simulink model "c00002M_harness"  (R2018a)
settings: Solver=FixedStepAuto  StartTime=0.0  StopTime=300  FixedStep=0.1  RelTol=1e-3
undefined symbols (not defined in the file): A1, hmax, R1, R2, sigbuilder_block, TempThreshold
(part 12 of 14)

== system c00002M_harness/M246/Tank3/Control ==
  note: 1: Maintenance
      | 2: Reference
      | 3: Manual
  ControlType : Inport
  ManualReference : Inport  Port=2
  EmergencyButton : Inport  Port=3
  Temperature : Inport  Port=4
  LiquidLevel : Inport  Port=5
  Constant : Constant  Value=0
  Constant1 : Constant  Value=TempThreshold
  Logical Operator : Logic  Operator=OR  AllPortsSameDT=off  OutDataTypeStr=boolean
  Logical Operator1 : Logic  Operator=OR  AllPortsSameDT=off  OutDataTypeStr=boolean
  ManualControlReference : Subsystem
  Relational Operator : RelationalOperator  Operator=>  OutDataTypeStr=boolean  RndMeth=Simplest
  Switch : Switch  Criteria=u2 > Threshold
  Switch1 : Switch  Criteria=u2 > Threshold
  LiquidIn : Outport
  LiquidOut : Outport  Port=2
  wires:
  ManualReference/1 -> ManualControlReference/1(ManualReference)
  LiquidLevel/1 -> ManualControlReference/2(LiquidLevel)
  Switch/1 -> LiquidIn/1
  Switch1/1 -> LiquidOut/1
  Constant/1 -> Switch1/1, Switch/1
  EmergencyButton/1 -> Logical Operator/1, Logical Operator1/1
  Relational Operator/1 -> Logical Operator1/2, Logical Operator/2
  Logical Operator/1 -> Switch1/2
  Logical Operator1/1 -> Switch/2
  Temperature/1 -> Relational Operator/1
  Constant1/1 -> Relational Operator/2
  ManualControlReference/1(LiquidIn) -> Switch/3
  ManualControlReference/2(LiquidOut) -> Switch1/3

== system c00002M_harness/M246/Tank3/TankModel ==
  LiquidIn : Inport
  LiquidOut : Inport  Port=2
  Add1 : Sum  Inputs=+-
  Constant1 : Constant  Value=0
  Constant2 : Constant  Value=0
  Constant3 : Constant
  Gain : Gain  Gain=1/R1
  Gain1 : Gain  Gain=1/A1
  Gain2 : Gain  Gain=1/R2
  Integrator : Integrator
  Saturation : Saturate  UpperLimit=hmax  LowerLimit=0
  Switch : Switch  Criteria=u2 ~= 0
  Switch1 : Switch  Criteria=u2 ~= 0
  LiquidLevel : Outport
  wires:
  Saturation/1 -> LiquidLevel/1, Gain2/1
  LiquidOut/1 -> Switch/2
  Add1/1 -> Gain1/1
  Gain2/1 -> Switch/1
  LiquidIn/1 -> Switch1/2
  Switch/1 -> Add1/2
  Switch1/1 -> Gain/1
  Constant2/1 -> Switch/3
  Constant3/1 -> Switch1/3
  Integrator/1 -> Saturation/1
  Gain1/1 -> Integrator/1
  Gain/1 -> Add1/1
  Constant1/1 -> Switch1/1

== system c00002M_harness/CPSUT/Tank1/Control/ManualControlReference ==
  ManualReference : Inport
  LiquidLevel : Inport  Port=2
  Add : Sum  Inputs=+-
  Add1 : Sum  Inputs=+-
  Gain1 : Gain  Gain=0.95
  Gain2 : Gain  Gain=0.95
  Relational Operator : RelationalOperator  Operator=>  OutDataTypeStr=boolean  RndMeth=Simplest
  Relational Operator1 : RelationalOperator  Operator=<  OutDataTypeStr=boolean  RndMeth=Simplest
  Saturation1 : Saturate  UpperLimit=hmax*0.9  LowerLimit=0
  LiquidIn : Outport
  LiquidOut : Outport  Port=2
  wires:
  LiquidLevel/1 -> Relational Operator/2, Add/1, Add1/1, Gain2/1
  Relational Operator/1 -> LiquidIn/1
  Relational Operator1/1 -> LiquidOut/1
  Add/1 -> Add1/2
  Add1/1 -> Relational Operator1/2
  Gain1/1 -> Saturation1/1
  Gain2/1 -> Add/2
  ManualReference/1 -> Gain1/1
  Saturation1/1 -> Relational Operator1/1, Relational Operator/1

== system c00002M_harness/CPSUT/Tank3/Control/ManualControlReference ==
  ManualReference : Inport
  LiquidLevel : Inport  Port=2
  Add : Sum  Inputs=+-
  Add1 : Sum  Inputs=+-
  Gain1 : Gain  Gain=0.95
  Gain2 : Gain  Gain=0.95
  Relational Operator : RelationalOperator  Operator=>  OutDataTypeStr=boolean  RndMeth=Simplest
  Relational Operator1 : RelationalOperator  Operator=<  OutDataTypeStr=boolean  RndMeth=Simplest
  Saturation1 : Saturate  UpperLimit=hmax*0.9  LowerLimit=0
  LiquidIn : Outport
  LiquidOut : Outport  Port=2
  wires:
  LiquidLevel/1 -> Relational Operator/2, Add/1, Add1/1, Gain2/1
  Relational Operator/1 -> LiquidIn/1
  Relational Operator1/1 -> LiquidOut/1
  Add/1 -> Add1/2
  Add1/1 -> Relational Operator1/2
  Gain1/1 -> Saturation1/1
  Gain2/1 -> Add/2
  ManualReference/1 -> Gain1/1
  Saturation1/1 -> Relational Operator1/1, Relational Operator/1

== system c00002M_harness/M001/Tank1/Control/ManualControlReference ==
  ManualReference : Inport
  LiquidLevel : Inport  Port=2
  Add : Sum  Inputs=+-
  Add1 : Sum  Inputs=+-
  Gain1 : Gain  Gain=0.95
  Gain2 : Gain  Gain=0.95
  Relational Operator : RelationalOperator  Operator=>  OutDataTypeStr=boolean  RndMeth=Simplest
  Relational Operator1 : RelationalOperator  Operator=<  OutDataTypeStr=boolean  RndMeth=Simplest
  Saturation1 : Saturate  UpperLimit=hmax*0.9  LowerLimit=0
  LiquidIn : Outport
  LiquidOut : Outport  Port=2
  wires:
  Saturation1/1 -> Relational Operator/1, Relational Operator1/1
  ManualReference/1 -> Gain1/1
  Gain2/1 -> Add/2
  Gain1/1 -> Saturation1/1
  Add1/1 -> Relational Operator1/2
  Add/1 -> Add1/2
  Relational Operator1/1 -> LiquidOut/1
  Relational Operator/1 -> LiquidIn/1
  LiquidLevel/1 -> Gain2/1, Add1/1, Add/1, Relational Operator/2

== system c00002M_harness/M001/Tank3/Control/ManualControlReference ==
  ManualReference : Inport
  LiquidLevel : Inport  Port=2
  Add : Sum  Inputs=+-
  Add1 : Sum  Inputs=+-
  Gain1 : Gain  Gain=0.95
  Gain2 : Gain  Gain=0.95
  Relational Operator : RelationalOperator  Operator=>  OutDataTypeStr=boolean  RndMeth=Simplest
  Relational Operator1 : RelationalOperator  Operator=<  OutDataTypeStr=boolean  RndMeth=Simplest
  Saturation1 : Saturate  UpperLimit=hmax*0.9  LowerLimit=0
  LiquidIn : Outport
  LiquidOut : Outport  Port=2
  wires:
  Saturation1/1 -> Relational Operator/1, Relational Operator1/1
  ManualReference/1 -> Gain1/1
  Gain2/1 -> Add/2
  Gain1/1 -> Saturation1/1
  Add1/1 -> Relational Operator1/2
  Add/1 -> Add1/2
  Relational Operator1/1 -> LiquidOut/1
  Relational Operator/1 -> LiquidIn/1
  LiquidLevel/1 -> Gain2/1, Add1/1, Add/1, Relational Operator/2

== system c00002M_harness/M002/Tank1/Control/ManualControlReference ==
  ManualReference : Inport
  LiquidLevel : Inport  Port=2
  Add : Sum  Inputs=+-
  Add1 : Sum  Inputs=+-
  Gain1 : Gain  Gain=0.95
  Gain2 : Gain  Gain=0.95
  Relational Operator : RelationalOperator  Operator=>  OutDataTypeStr=boolean  RndMeth=Simplest
  Relational Operator1 : RelationalOperator  Operator=<  OutDataTypeStr=boolean  RndMeth=Simplest
  Saturation1 : Saturate  UpperLimit=hmax*0.9  LowerLimit=0
  LiquidIn : Outport
  LiquidOut : Outport  Port=2
  wires:
  LiquidLevel/1 -> Relational Operator/2, Add/1, Add1/1, Gain2/1
  Relational Operator/1 -> LiquidIn/1
  Relational Operator1/1 -> LiquidOut/1
  Add/1 -> Add1/2
  Add1/1 -> Relational Operator1/2
  Gain1/1 -> Saturation1/1
  Gain2/1 -> Add/2
  ManualReference/1 -> Gain1/1
  Saturation1/1 -> Relational Operator1/1, Relational Operator/1

== system c00002M_harness/M002/Tank3/Control/ManualControlReference ==
  ManualReference : Inport
  LiquidLevel : Inport  Port=2
  Add : Sum  Inputs=+-
  Add1 : Sum  Inputs=+-
  Gain1 : Gain  Gain=0.95
  Gain2 : Gain  Gain=0.95
  Relational Operator : RelationalOperator  Operator=>  OutDataTypeStr=boolean  RndMeth=Simplest
  Relational Operator1 : RelationalOperator  Operator=<  OutDataTypeStr=boolean  RndMeth=Simplest
  Saturation1 : Saturate  UpperLimit=hmax*0.9  LowerLimit=0
  LiquidIn : Outport
  LiquidOut : Outport  Port=2
  wires:
  LiquidLevel/1 -> Relational Operator/2, Add/1, Add1/1, Gain2/1
  Relational Operator/1 -> LiquidIn/1
  Relational Operator1/1 -> LiquidOut/1
  Add/1 -> Add1/2
  Add1/1 -> Relational Operator1/2
  Gain1/1 -> Saturation1/1
  Gain2/1 -> Add/2
  ManualReference/1 -> Gain1/1
  Saturation1/1 -> Relational Operator1/1, Relational Operator/1

== system c00002M_harness/M003/Tank1/Control/ManualControlReference ==
  ManualReference : Inport
  LiquidLevel : Inport  Port=2
  Add : Sum  Inputs=+-
  Add1 : Sum  Inputs=+-
  Gain1 : Gain  Gain=0.95
  Gain2 : Gain  Gain=0.95
  Relational Operator : RelationalOperator  Operator=>  OutDataTypeStr=boolean  RndMeth=Simplest
  Relational Operator1 : RelationalOperator  Operator=<  OutDataTypeStr=boolean  RndMeth=Simplest
  Saturation1 : Saturate  UpperLimit=hmax*0.9  LowerLimit=0
  LiquidIn : Outport
  LiquidOut : Outport  Port=2
  wires:
  LiquidLevel/1 -> Relational Operator/2, Add/1, Add1/1, Gain2/1
  Relational Operator/1 -> LiquidIn/1
  Relational Operator1/1 -> LiquidOut/1
  Add/1 -> Add1/2
  Add1/1 -> Relational Operator1/2
  Gain1/1 -> Saturation1/1
  Gain2/1 -> Add/2
  ManualReference/1 -> Gain1/1
  Saturation1/1 -> Relational Operator1/1, Relational Operator/1

== system c00002M_harness/M003/Tank3/Control/ManualControlReference ==
  ManualReference : Inport
  LiquidLevel : Inport  Port=2
  Add : Sum  Inputs=+-
  Add1 : Sum  Inputs=+-
  Gain1 : Gain  Gain=0.95
  Gain2 : Gain  Gain=0.95
  Relational Operator : RelationalOperator  Operator=>  OutDataTypeStr=boolean  RndMeth=Simplest
  Relational Operator1 : RelationalOperator  Operator=<  OutDataTypeStr=boolean  RndMeth=Simplest
  Saturation1 : Saturate  UpperLimit=hmax*0.9  LowerLimit=0
  LiquidIn : Outport
  LiquidOut : Outport  Port=2
  wires:
  LiquidLevel/1 -> Relational Operator/2, Add/1, Add1/1, Gain2/1
  Relational Operator/1 -> LiquidIn/1
  Relational Operator1/1 -> LiquidOut/1
  Add/1 -> Add1/2
  Add1/1 -> Relational Operator1/2
  Gain1/1 -> Saturation1/1
  Gain2/1 -> Add/2
  ManualReference/1 -> Gain1/1
  Saturation1/1 -> Relational Operator1/1, Relational Operator/1

== system c00002M_harness/M004/Tank1/Control/ManualControlReference ==
  ManualReference : Inport
  LiquidLevel : Inport  Port=2
  Add : Sum  Inputs=+-
  Add1 : Sum  Inputs=+-
  Gain1 : Gain  Gain=0.95
  Gain2 : Gain  Gain=0.95
  Relational Operator : RelationalOperator  Operator=>  OutDataTypeStr=boolean  RndMeth=Simplest
  Relational Operator1 : RelationalOperator  Operator=<  OutDataTypeStr=boolean  RndMeth=Simplest
  Saturation1 : Saturate  UpperLimit=hmax*0.9  LowerLimit=0
  LiquidIn : Outport
  LiquidOut : Outport  Port=2
  wires:
  LiquidLevel/1 -> Relational Operator/2, Add/1, Add1/1, Gain2/1
  Relational Operator/1 -> LiquidIn/1
  Relational Operator1/1 -> LiquidOut/1
  Add/1 -> Add1/2
  Add1/1 -> Relational Operator1/2
  Gain1/1 -> Saturation1/1
  Gain2/1 -> Add/2
  ManualReference/1 -> Gain1/1
  Saturation1/1 -> Relational Operator1/1, Relational Operator/1

== system c00002M_harness/M004/Tank3/Control/ManualControlReference ==
  ManualReference : Inport
  LiquidLevel : Inport  Port=2
  Add : Sum  Inputs=+-
  Add1 : Sum  Inputs=+-
  Gain1 : Gain  Gain=0.95
  Gain2 : Gain  Gain=0.95
  Relational Operator : RelationalOperator  Operator=>  OutDataTypeStr=boolean  RndMeth=Simplest
  Relational Operator1 : RelationalOperator  Operator=<  OutDataTypeStr=boolean  RndMeth=Simplest
  Saturation1 : Saturate  UpperLimit=hmax*0.9  LowerLimit=0
  LiquidIn : Outport
  LiquidOut : Outport  Port=2
  wires:
  LiquidLevel/1 -> Relational Operator/2, Add/1, Add1/1, Gain2/1
  Relational Operator/1 -> LiquidIn/1
  Relational Operator1/1 -> LiquidOut/1
  Add/1 -> Add1/2
  Add1/1 -> Relational Operator1/2
  Gain1/1 -> Saturation1/1
  Gain2/1 -> Add/2
  ManualReference/1 -> Gain1/1
  Saturation1/1 -> Relational Operator1/1, Relational Operator/1

== system c00002M_harness/M046/Tank1/Control/ManualControlReference ==
  ManualReference : Inport
  LiquidLevel : Inport  Port=2
  Add : Sum
  Add1 : Sum  Inputs=+-
  Gain1 : Gain  Gain=0.95
  Gain2 : Gain  Gain=0.95
  Relational Operator : RelationalOperator  Operator=>  OutDataTypeStr=boolean  RndMeth=Simplest
  Relational Operator1 : RelationalOperator  Operator=<  OutDataTypeStr=boolean  RndMeth=Simplest
  Saturation1 : Saturate  UpperLimit=hmax*0.9  LowerLimit=0
  LiquidIn : Outport
  LiquidOut : Outport  Port=2
  wires:
  LiquidLevel/1 -> Relational Operator/2, Add/1, Add1/1, Gain2/1
  Relational Operator/1 -> LiquidIn/1
  Relational Operator1/1 -> LiquidOut/1
  Add/1 -> Add1/2
  Add1/1 -> Relational Operator1/2
  Gain1/1 -> Saturation1/1
  Gain2/1 -> Add/2
  ManualReference/1 -> Gain1/1
  Saturation1/1 -> Relational Operator1/1, Relational Operator/1

== system c00002M_harness/M046/Tank3/Control/ManualControlReference ==
  ManualReference : Inport
  LiquidLevel : Inport  Port=2
  Add : Sum  Inputs=+-
  Add1 : Sum  Inputs=+-
  Gain1 : Gain  Gain=0.95
  Gain2 : Gain  Gain=0.95
  Relational Operator : RelationalOperator  Operator=>  OutDataTypeStr=boolean  RndMeth=Simplest
  Relational Operator1 : RelationalOperator  Operator=<  OutDataTypeStr=boolean  RndMeth=Simplest
  Saturation1 : Saturate  UpperLimit=hmax*0.9  LowerLimit=0
  LiquidIn : Outport
  LiquidOut : Outport  Port=2
  wires:
  LiquidLevel/1 -> Relational Operator/2, Add/1, Add1/1, Gain2/1
  Relational Operator/1 -> LiquidIn/1
  Relational Operator1/1 -> LiquidOut/1
  Add/1 -> Add1/2
  Add1/1 -> Relational Operator1/2
  Gain1/1 -> Saturation1/1
  Gain2/1 -> Add/2
  ManualReference/1 -> Gain1/1
  Saturation1/1 -> Relational Operator1/1, Relational Operator/1

== system c00002M_harness/M047/Tank1/Control/ManualControlReference ==
  ManualReference : Inport
  LiquidLevel : Inport  Port=2
  Add : Sum  Inputs=--
  Add1 : Sum  Inputs=+-
  Gain1 : Gain  Gain=0.95
  Gain2 : Gain  Gain=0.95
  Relational Operator : RelationalOperator  Operator=>  OutDataTypeStr=boolean  RndMeth=Simplest
  Relational Operator1 : RelationalOperator  Operator=<  OutDataTypeStr=boolean  RndMeth=Simplest
  Saturation1 : Saturate  UpperLimit=hmax*0.9  LowerLimit=0
  LiquidIn : Outport
  LiquidOut : Outport  Port=2
  wires:
  LiquidLevel/1 -> Relational Operator/2, Add/1, Add1/1, Gain2/1
  Relational Operator/1 -> LiquidIn/1
  Relational Operator1/1 -> LiquidOut/1
  Add/1 -> Add1/2
  Add1/1 -> Relational Operator1/2
  Gain1/1 -> Saturation1/1
  Gain2/1 -> Add/2
  ManualReference/1 -> Gain1/1
  Saturation1/1 -> Relational Operator1/1, Relational Operator/1

== system c00002M_harness/M047/Tank3/Control/ManualControlReference ==
  ManualReference : Inport
  LiquidLevel : Inport  Port=2
  Add : Sum  Inputs=+-
  Add1 : Sum  Inputs=+-
  Gain1 : Gain  Gain=0.95
  Gain2 : Gain  Gain=0.95
  Relational Operator : RelationalOperator  Operator=>  OutDataTypeStr=boolean  RndMeth=Simplest
  Relational Operator1 : RelationalOperator  Operator=<  OutDataTypeStr=boolean  RndMeth=Simplest
  Saturation1 : Saturate  UpperLimit=hmax*0.9  LowerLimit=0
  LiquidIn : Outport
  LiquidOut : Outport  Port=2
  wires:
  LiquidLevel/1 -> Relational Operator/2, Add/1, Add1/1, Gain2/1
  Relational Operator/1 -> LiquidIn/1
  Relational Operator1/1 -> LiquidOut/1
  Add/1 -> Add1/2
  Add1/1 -> Relational Operator1/2
  Gain1/1 -> Saturation1/1
  Gain2/1 -> Add/2
  ManualReference/1 -> Gain1/1
  Saturation1/1 -> Relational Operator1/1, Relational Operator/1

== system c00002M_harness/M048/Tank1/Control/ManualControlReference ==
  ManualReference : Inport
  LiquidLevel : Inport  Port=2
  Add : Sum  Inputs=-+
  Add1 : Sum  Inputs=+-
  Gain1 : Gain  Gain=0.95
  Gain2 : Gain  Gain=0.95
  Relational Operator : RelationalOperator  Operator=>  OutDataTypeStr=boolean  RndMeth=Simplest
  Relational Operator1 : RelationalOperator  Operator=<  OutDataTypeStr=boolean  RndMeth=Simplest
  Saturation1 : Saturate  UpperLimit=hmax*0.9  LowerLimit=0
  LiquidIn : Outport
  LiquidOut : Outport  Port=2
  wires:
  LiquidLevel/1 -> Relational Operator/2, Add/1, Add1/1, Gain2/1
  Relational Operator/1 -> LiquidIn/1
  Relational Operator1/1 -> LiquidOut/1
  Add/1 -> Add1/2
  Add1/1 -> Relational Operator1/2
  Gain1/1 -> Saturation1/1
  Gain2/1 -> Add/2
  ManualReference/1 -> Gain1/1
  Saturation1/1 -> Relational Operator1/1, Relational Operator/1

== system c00002M_harness/M048/Tank3/Control/ManualControlReference ==
  ManualReference : Inport
  LiquidLevel : Inport  Port=2
  Add : Sum  Inputs=+-
  Add1 : Sum  Inputs=+-
  Gain1 : Gain  Gain=0.95
  Gain2 : Gain  Gain=0.95
  Relational Operator : RelationalOperator  Operator=>  OutDataTypeStr=boolean  RndMeth=Simplest
  Relational Operator1 : RelationalOperator  Operator=<  OutDataTypeStr=boolean  RndMeth=Simplest
  Saturation1 : Saturate  UpperLimit=hmax*0.9  LowerLimit=0
  LiquidIn : Outport
  LiquidOut : Outport  Port=2
  wires:
  LiquidLevel/1 -> Relational Operator/2, Add/1, Add1/1, Gain2/1
  Relational Operator/1 -> LiquidIn/1
  Relational Operator1/1 -> LiquidOut/1
  Add/1 -> Add1/2
  Add1/1 -> Relational Operator1/2
  Gain1/1 -> Saturation1/1
  Gain2/1 -> Add/2
  ManualReference/1 -> Gain1/1
  Saturation1/1 -> Relational Operator1/1, Relational Operator/1

== system c00002M_harness/M049/Tank1/Control/ManualControlReference ==
  ManualReference : Inport
  LiquidLevel : Inport  Port=2
  Add : Sum  Inputs=+-
  Add1 : Sum
  Gain1 : Gain  Gain=0.95
  Gain2 : Gain  Gain=0.95
  Relational Operator : RelationalOperator  Operator=>  OutDataTypeStr=boolean  RndMeth=Simplest
  Relational Operator1 : RelationalOperator  Operator=<  OutDataTypeStr=boolean  RndMeth=Simplest
  Saturation1 : Saturate  UpperLimit=hmax*0.9  LowerLimit=0
  LiquidIn : Outport
  LiquidOut : Outport  Port=2
  wires:
  LiquidLevel/1 -> Relational Operator/2, Add/1, Add1/1, Gain2/1
  Relational Operator/1 -> LiquidIn/1
  Relational Operator1/1 -> LiquidOut/1
  Add/1 -> Add1/2
  Add1/1 -> Relational Operator1/2
  Gain1/1 -> Saturation1/1
  Gain2/1 -> Add/2
  ManualReference/1 -> Gain1/1
  Saturation1/1 -> Relational Operator1/1, Relational Operator/1

== system c00002M_harness/M049/Tank3/Control/ManualControlReference ==
  ManualReference : Inport
  LiquidLevel : Inport  Port=2
  Add : Sum  Inputs=+-
  Add1 : Sum  Inputs=+-
  Gain1 : Gain  Gain=0.95
  Gain2 : Gain  Gain=0.95
  Relational Operator : RelationalOperator  Operator=>  OutDataTypeStr=boolean  RndMeth=Simplest
  Relational Operator1 : RelationalOperator  Operator=<  OutDataTypeStr=boolean  RndMeth=Simplest
  Saturation1 : Saturate  UpperLimit=hmax*0.9  LowerLimit=0
  LiquidIn : Outport
  LiquidOut : Outport  Port=2
  wires:
  LiquidLevel/1 -> Relational Operator/2, Add/1, Add1/1, Gain2/1
  Relational Operator/1 -> LiquidIn/1
  Relational Operator1/1 -> LiquidOut/1
  Add/1 -> Add1/2
  Add1/1 -> Relational Operator1/2
  Gain1/1 -> Saturation1/1
  Gain2/1 -> Add/2
  ManualReference/1 -> Gain1/1
  Saturation1/1 -> Relational Operator1/1, Relational Operator/1

== system c00002M_harness/M050/Tank1/Control/ManualControlReference ==
  ManualReference : Inport
  LiquidLevel : Inport  Port=2
  Add : Sum  Inputs=+-
  Add1 : Sum  Inputs=--
  Gain1 : Gain  Gain=0.95
  Gain2 : Gain  Gain=0.95
  Relational Operator : RelationalOperator  Operator=>  OutDataTypeStr=boolean  RndMeth=Simplest
  Relational Operator1 : RelationalOperator  Operator=<  OutDataTypeStr=boolean  RndMeth=Simplest
  Saturation1 : Saturate  UpperLimit=hmax*0.9  LowerLimit=0
  LiquidIn : Outport
  LiquidOut : Outport  Port=2
  wires:
  LiquidLevel/1 -> Relational Operator/2, Add/1, Add1/1, Gain2/1
  Relational Operator/1 -> LiquidIn/1
  Relational Operator1/1 -> LiquidOut/1
  Add/1 -> Add1/2
  Add1/1 -> Relational Operator1/2
  Gain1/1 -> Saturation1/1
  Gain2/1 -> Add/2
  ManualReference/1 -> Gain1/1
  Saturation1/1 -> Relational Operator1/1, Relational Operator/1

== system c00002M_harness/M050/Tank3/Control/ManualControlReference ==
  ManualReference : Inport
  LiquidLevel : Inport  Port=2
  Add : Sum  Inputs=+-
  Add1 : Sum  Inputs=+-
  Gain1 : Gain  Gain=0.95
  Gain2 : Gain  Gain=0.95
  Relational Operator : RelationalOperator  Operator=>  OutDataTypeStr=boolean  RndMeth=Simplest
  Relational Operator1 : RelationalOperator  Operator=<  OutDataTypeStr=boolean  RndMeth=Simplest
  Saturation1 : Saturate  UpperLimit=hmax*0.9  LowerLimit=0
  LiquidIn : Outport
  LiquidOut : Outport  Port=2
  wires:
  LiquidLevel/1 -> Relational Operator/2, Add/1, Add1/1, Gain2/1
  Relational Operator/1 -> LiquidIn/1
  Relational Operator1/1 -> LiquidOut/1
  Add/1 -> Add1/2
  Add1/1 -> Relational Operator1/2
  Gain1/1 -> Saturation1/1
  Gain2/1 -> Add/2
  ManualReference/1 -> Gain1/1
  Saturation1/1 -> Relational Operator1/1, Relational Operator/1

== system c00002M_harness/M051/Tank1/Control/ManualControlReference ==
  ManualReference : Inport
  LiquidLevel : Inport  Port=2
  Add : Sum  Inputs=+-
  Add1 : Sum  Inputs=-+
  Gain1 : Gain  Gain=0.95
  Gain2 : Gain  Gain=0.95
  Relational Operator : RelationalOperator  Operator=>  OutDataTypeStr=boolean  RndMeth=Simplest
  Relational Operator1 : RelationalOperator  Operator=<  OutDataTypeStr=boolean  RndMeth=Simplest
  Saturation1 : Saturate  UpperLimit=hmax*0.9  LowerLimit=0
  LiquidIn : Outport
  LiquidOut : Outport  Port=2
  wires:
  LiquidLevel/1 -> Relational Operator/2, Add/1, Add1/1, Gain2/1
  Relational Operator/1 -> LiquidIn/1
  Relational Operator1/1 -> LiquidOut/1
  Add/1 -> Add1/2
  Add1/1 -> Relational Operator1/2
  Gain1/1 -> Saturation1/1
  Gain2/1 -> Add/2
  ManualReference/1 -> Gain1/1
  Saturation1/1 -> Relational Operator1/1, Relational Operator/1

== system c00002M_harness/M051/Tank3/Control/ManualControlReference ==
  ManualReference : Inport
  LiquidLevel : Inport  Port=2
  Add : Sum  Inputs=+-
  Add1 : Sum  Inputs=+-
  Gain1 : Gain  Gain=0.95
  Gain2 : Gain  Gain=0.95
  Relational Operator : RelationalOperator  Operator=>  OutDataTypeStr=boolean  RndMeth=Simplest
  Relational Operator1 : RelationalOperator  Operator=<  OutDataTypeStr=boolean  RndMeth=Simplest
  Saturation1 : Saturate  UpperLimit=hmax*0.9  LowerLimit=0
  LiquidIn : Outport
  LiquidOut : Outport  Port=2
  wires:
  LiquidLevel/1 -> Relational Operator/2, Add/1, Add1/1, Gain2/1
  Relational Operator/1 -> LiquidIn/1
  Relational Operator1/1 -> LiquidOut/1
  Add/1 -> Add1/2
  Add1/1 -> Relational Operator1/2
  Gain1/1 -> Saturation1/1
  Gain2/1 -> Add/2
  ManualReference/1 -> Gain1/1
  Saturation1/1 -> Relational Operator1/1, Relational Operator/1

== system c00002M_harness/M052/Tank1/Control/ManualControlReference ==
  ManualReference : Inport
  LiquidLevel : Inport  Port=2
  Add : Sum  Inputs=+-
  Add1 : Sum  Inputs=+-
  Gain1 : Gain  Gain=0.90
  Gain2 : Gain  Gain=0.95
  Relational Operator : RelationalOperator  Operator=>  OutDataTypeStr=boolean  RndMeth=Simplest
  Relational Operator1 : RelationalOperator  Operator=<  OutDataTypeStr=boolean  RndMeth=Simplest
  Saturation1 : Saturate  UpperLimit=hmax*0.9  LowerLimit=0
  LiquidIn : Outport
  LiquidOut : Outport  Port=2
  wires:
  LiquidLevel/1 -> Relational Operator/2, Add/1, Add1/1, Gain2/1
  Relational Operator/1 -> LiquidIn/1
  Relational Operator1/1 -> LiquidOut/1
  Add/1 -> Add1/2
  Add1/1 -> Relational Operator1/2
  Gain1/1 -> Saturation1/1
  Gain2/1 -> Add/2
  ManualReference/1 -> Gain1/1
  Saturation1/1 -> Relational Operator1/1, Relational Operator/1

== system c00002M_harness/M052/Tank3/Control/ManualControlReference ==
  ManualReference : Inport
  LiquidLevel : Inport  Port=2
  Add : Sum  Inputs=+-
  Add1 : Sum  Inputs=+-
  Gain1 : Gain  Gain=0.95
  Gain2 : Gain  Gain=0.95
  Relational Operator : RelationalOperator  Operator=>  OutDataTypeStr=boolean  RndMeth=Simplest
  Relational Operator1 : RelationalOperator  Operator=<  OutDataTypeStr=boolean  RndMeth=Simplest
  Saturation1 : Saturate  UpperLimit=hmax*0.9  LowerLimit=0
  LiquidIn : Outport
  LiquidOut : Outport  Port=2
  wires:
  LiquidLevel/1 -> Relational Operator/2, Add/1, Add1/1, Gain2/1
  Relational Operator/1 -> LiquidIn/1
  Relational Operator1/1 -> LiquidOut/1
  Add/1 -> Add1/2
  Add1/1 -> Relational Operator1/2
  Gain1/1 -> Saturation1/1
  Gain2/1 -> Add/2
  ManualReference/1 -> Gain1/1
  Saturation1/1 -> Relational Operator1/1, Relational Operator/1

== system c00002M_harness/M053/Tank1/Control/ManualControlReference ==
  ManualReference : Inport
  LiquidLevel : Inport  Port=2
  Add : Sum  Inputs=+-
  Add1 : Sum  Inputs=+-
  Gain1 : Gain  Gain=0.95
  Gain2 : Gain  Gain=0.90
  Relational Operator : RelationalOperator  Operator=>  OutDataTypeStr=boolean  RndMeth=Simplest
  Relational Operator1 : RelationalOperator  Operator=<  OutDataTypeStr=boolean  RndMeth=Simplest
  Saturation1 : Saturate  UpperLimit=hmax*0.9  LowerLimit=0
  LiquidIn : Outport
  LiquidOut : Outport  Port=2
  wires:
  LiquidLevel/1 -> Relational Operator/2, Add/1, Add1/1, Gain2/1
  Relational Operator/1 -> LiquidIn/1
  Relational Operator1/1 -> LiquidOut/1
  Add/1 -> Add1/2
  Add1/1 -> Relational Operator1/2
  Gain1/1 -> Saturation1/1
  Gain2/1 -> Add/2
  ManualReference/1 -> Gain1/1
  Saturation1/1 -> Relational Operator1/1, Relational Operator/1

== system c00002M_harness/M053/Tank3/Control/ManualControlReference ==
  ManualReference : Inport
  LiquidLevel : Inport  Port=2
  Add : Sum  Inputs=+-
  Add1 : Sum  Inputs=+-
  Gain1 : Gain  Gain=0.95
  Gain2 : Gain  Gain=0.95
  Relational Operator : RelationalOperator  Operator=>  OutDataTypeStr=boolean  RndMeth=Simplest
  Relational Operator1 : RelationalOperator  Operator=<  OutDataTypeStr=boolean  RndMeth=Simplest
  Saturation1 : Saturate  UpperLimit=hmax*0.9  LowerLimit=0
  LiquidIn : Outport
  LiquidOut : Outport  Port=2
  wires:
  LiquidLevel/1 -> Relational Operator/2, Add/1, Add1/1, Gain2/1
  Relational Operator/1 -> LiquidIn/1
  Relational Operator1/1 -> LiquidOut/1
  Add/1 -> Add1/2
  Add1/1 -> Relational Operator1/2
  Gain1/1 -> Saturation1/1
  Gain2/1 -> Add/2
  ManualReference/1 -> Gain1/1
  Saturation1/1 -> Relational Operator1/1, Relational Operator/1

== system c00002M_harness/M054/Tank1/Control/ManualControlReference ==
  ManualReference : Inport
  LiquidLevel : Inport  Port=2
  Add : Sum  Inputs=+-
  Add1 : Sum  Inputs=+-
  Gain1 : Gain  Gain=0.95
  Gain2 : Gain  Gain=0.95
  Relational Operator : RelationalOperator  Operator=<  OutDataTypeStr=boolean  RndMeth=Simplest
  Relational Operator1 : RelationalOperator  Operator=<  OutDataTypeStr=boolean  RndMeth=Simplest
  Saturation1 : Saturate  UpperLimit=hmax*0.9  LowerLimit=0
  LiquidIn : Outport
  LiquidOut : Outport  Port=2
  wires:
  LiquidLevel/1 -> Relational Operator/2, Add/1, Add1/1, Gain2/1
  Relational Operator/1 -> LiquidIn/1
  Relational Operator1/1 -> LiquidOut/1
  Add/1 -> Add1/2
  Add1/1 -> Relational Operator1/2
  Gain1/1 -> Saturation1/1
  Gain2/1 -> Add/2
  ManualReference/1 -> Gain1/1
  Saturation1/1 -> Relational Operator1/1, Relational Operator/1

== system c00002M_harness/M054/Tank3/Control/ManualControlReference ==
  ManualReference : Inport
  LiquidLevel : Inport  Port=2
  Add : Sum  Inputs=+-
  Add1 : Sum  Inputs=+-
  Gain1 : Gain  Gain=0.95
  Gain2 : Gain  Gain=0.95
  Relational Operator : RelationalOperator  Operator=>  OutDataTypeStr=boolean  RndMeth=Simplest
  Relational Operator1 : RelationalOperator  Operator=<  OutDataTypeStr=boolean  RndMeth=Simplest
  Saturation1 : Saturate  UpperLimit=hmax*0.9  LowerLimit=0
  LiquidIn : Outport
  LiquidOut : Outport  Port=2
  wires:
  LiquidLevel/1 -> Relational Operator/2, Add/1, Add1/1, Gain2/1
  Relational Operator/1 -> LiquidIn/1
  Relational Operator1/1 -> LiquidOut/1
  Add/1 -> Add1/2
  Add1/1 -> Relational Operator1/2
  Gain1/1 -> Saturation1/1
  Gain2/1 -> Add/2
  ManualReference/1 -> Gain1/1
  Saturation1/1 -> Relational Operator1/1, Relational Operator/1

== system c00002M_harness/M055/Tank1/Control/ManualControlReference ==
  ManualReference : Inport
  LiquidLevel : Inport  Port=2
  Add : Sum  Inputs=+-
  Add1 : Sum  Inputs=+-
  Gain1 : Gain  Gain=0.95
  Gain2 : Gain  Gain=0.95
  Relational Operator : RelationalOperator  Operator=>  OutDataTypeStr=boolean  RndMeth=Simplest
  Relational Operator1 : RelationalOperator  Operator=>  OutDataTypeStr=boolean  RndMeth=Simplest
  Saturation1 : Saturate  UpperLimit=hmax*0.9  LowerLimit=0
  LiquidIn : Outport
  LiquidOut : Outport  Port=2
  wires:
  LiquidLevel/1 -> Relational Operator/2, Add/1, Add1/1, Gain2/1
  Relational Operator/1 -> LiquidIn/1
  Relational Operator1/1 -> LiquidOut/1
  Add/1 -> Add1/2
  Add1/1 -> Relational Operator1/2
  Gain1/1 -> Saturation1/1
  Gain2/1 -> Add/2
  ManualReference/1 -> Gain1/1
  Saturation1/1 -> Relational Operator1/1, Relational Operator/1

== system c00002M_harness/M055/Tank3/Control/ManualControlReference ==
  ManualReference : Inport
  LiquidLevel : Inport  Port=2
  Add : Sum  Inputs=+-
  Add1 : Sum  Inputs=+-
  Gain1 : Gain  Gain=0.95
  Gain2 : Gain  Gain=0.95
  Relational Operator : RelationalOperator  Operator=>  OutDataTypeStr=boolean  RndMeth=Simplest
  Relational Operator1 : RelationalOperator  Operator=<  OutDataTypeStr=boolean  RndMeth=Simplest
  Saturation1 : Saturate  UpperLimit=hmax*0.9  LowerLimit=0
  LiquidIn : Outport
  LiquidOut : Outport  Port=2
  wires:
  LiquidLevel/1 -> Relational Operator/2, Add/1, Add1/1, Gain2/1
  Relational Operator/1 -> LiquidIn/1
  Relational Operator1/1 -> LiquidOut/1
  Add/1 -> Add1/2
  Add1/1 -> Relational Operator1/2
  Gain1/1 -> Saturation1/1
  Gain2/1 -> Add/2
  ManualReference/1 -> Gain1/1
  Saturation1/1 -> Relational Operator1/1, Relational Operator/1

== system c00002M_harness/M056/Tank1/Control/ManualControlReference ==
  ManualReference : Inport
  LiquidLevel : Inport  Port=2
  Add : Sum  Inputs=+-
  Add1 : Sum  Inputs=+-
  Gain1 : Gain  Gain=0.95
  Gain2 : Gain  Gain=0.95
  Relational Operator : RelationalOperator  Operator=>  OutDataTypeStr=boolean  RndMeth=Simplest
  Relational Operator1 : RelationalOperator  Operator=<  OutDataTypeStr=boolean  RndMeth=Simplest
  Saturation1 : Saturate  UpperLimit=(hmax+1)*0.9  LowerLimit=0
  LiquidIn : Outport
  LiquidOut : Outport  Port=2
  wires:
  LiquidLevel/1 -> Relational Operator/2, Add/1, Add1/1, Gain2/1
  Relational Operator/1 -> LiquidIn/1
  Relational Operator1/1 -> LiquidOut/1
  Add/1 -> Add1/2
  Add1/1 -> Relational Operator1/2
  Gain1/1 -> Saturation1/1
  Gain2/1 -> Add/2
  ManualReference/1 -> Gain1/1
  Saturation1/1 -> Relational Operator1/1, Relational Operator/1

== system c00002M_harness/M056/Tank3/Control/ManualControlReference ==
  ManualReference : Inport
  LiquidLevel : Inport  Port=2
  Add : Sum  Inputs=+-
  Add1 : Sum  Inputs=+-
  Gain1 : Gain  Gain=0.95
  Gain2 : Gain  Gain=0.95
  Relational Operator : RelationalOperator  Operator=>  OutDataTypeStr=boolean  RndMeth=Simplest
  Relational Operator1 : RelationalOperator  Operator=<  OutDataTypeStr=boolean  RndMeth=Simplest
  Saturation1 : Saturate  UpperLimit=hmax*0.9  LowerLimit=0
  LiquidIn : Outport
  LiquidOut : Outport  Port=2
  wires:
  LiquidLevel/1 -> Relational Operator/2, Add/1, Add1/1, Gain2/1
  Relational Operator/1 -> LiquidIn/1
  Relational Operator1/1 -> LiquidOut/1
  Add/1 -> Add1/2
  Add1/1 -> Relational Operator1/2
  Gain1/1 -> Saturation1/1
  Gain2/1 -> Add/2
  ManualReference/1 -> Gain1/1
  Saturation1/1 -> Relational Operator1/1, Relational Operator/1

== system c00002M_harness/M057/Tank1/Control/ManualControlReference ==
  ManualReference : Inport
  LiquidLevel : Inport  Port=2
  Add : Sum  Inputs=+-
  Add1 : Sum  Inputs=+-
  Gain1 : Gain  Gain=0.95
  Gain2 : Gain  Gain=0.95
  Relational Operator : RelationalOperator  Operator=>  OutDataTypeStr=boolean  RndMeth=Simplest
  Relational Operator1 : RelationalOperator  Operator=<  OutDataTypeStr=boolean  RndMeth=Simplest
  Saturation1 : Saturate  UpperLimit=hmax*0.9  LowerLimit=0
  LiquidIn : Outport
  LiquidOut : Outport  Port=2
  wires:
  LiquidLevel/1 -> Relational Operator/2, Add/1, Add1/1, Gain2/1
  Relational Operator/1 -> LiquidIn/1
  Relational Operator1/1 -> LiquidOut/1
  Add/1 -> Add1/2
  Add1/1 -> Relational Operator1/2
  Gain1/1 -> Saturation1/1
  Gain2/1 -> Add/2
  ManualReference/1 -> Gain1/1
  Saturation1/1 -> Relational Operator1/1, Relational Operator/1

== system c00002M_harness/M057/Tank3/Control/ManualControlReference ==
  ManualReference : Inport
  LiquidLevel : Inport  Port=2
  Add : Sum  Inputs=+-
  Add1 : Sum  Inputs=+-
  Gain1 : Gain  Gain=0.95
  Gain2 : Gain  Gain=0.95
  Relational Operator : RelationalOperator  Operator=>  OutDataTypeStr=boolean  RndMeth=Simplest
  Relational Operator1 : RelationalOperator  Operator=<  OutDataTypeStr=boolean  RndMeth=Simplest
  Saturation1 : Saturate  UpperLimit=hmax*0.9  LowerLimit=0
  LiquidIn : Outport
  LiquidOut : Outport  Port=2
  wires:
  LiquidLevel/1 -> Relational Operator/2, Add/1, Add1/1, Gain2/1
  Relational Operator/1 -> LiquidIn/1
  Relational Operator1/1 -> LiquidOut/1
  Add/1 -> Add1/2
  Add1/1 -> Relational Operator1/2
  Gain1/1 -> Saturation1/1
  Gain2/1 -> Add/2
  ManualReference/1 -> Gain1/1
  Saturation1/1 -> Relational Operator1/1, Relational Operator/1

== system c00002M_harness/M058/Tank1/Control/ManualControlReference ==
  ManualReference : Inport
  LiquidLevel : Inport  Port=2
  Add : Sum  Inputs=+-
  Add1 : Sum  Inputs=+-
  Gain1 : Gain  Gain=0.95
  Gain2 : Gain  Gain=0.95
  Relational Operator : RelationalOperator  Operator=>  OutDataTypeStr=boolean  RndMeth=Simplest
  Relational Operator1 : RelationalOperator  Operator=<  OutDataTypeStr=boolean  RndMeth=Simplest
  Saturation1 : Saturate  UpperLimit=hmax*0.9  LowerLimit=0
  LiquidIn : Outport
  LiquidOut : Outport  Port=2
  wires:
  LiquidLevel/1 -> Relational Operator/2, Add/1, Add1/1, Gain2/1
  Relational Operator/1 -> LiquidIn/1
  Relational Operator1/1 -> LiquidOut/1
  Add/1 -> Add1/2
  Add1/1 -> Relational Operator1/2
  Gain1/1 -> Saturation1/1
  Gain2/1 -> Add/2
  ManualReference/1 -> Gain1/1
  Saturation1/1 -> Relational Operator1/1, Relational Operator/1

== system c00002M_harness/M058/Tank3/Control/ManualControlReference ==
  ManualReference : Inport
  LiquidLevel : Inport  Port=2
  Add : Sum  Inputs=+-
  Add1 : Sum  Inputs=+-
  Gain1 : Gain  Gain=0.95
  Gain2 : Gain  Gain=0.95
  Relational Operator : RelationalOperator  Operator=>  OutDataTypeStr=boolean  RndMeth=Simplest
  Relational Operator1 : RelationalOperator  Operator=<  OutDataTypeStr=boolean  RndMeth=Simplest
  Saturation1 : Saturate  UpperLimit=hmax*0.9  LowerLimit=0
  LiquidIn : Outport
  LiquidOut : Outport  Port=2
  wires:
  LiquidLevel/1 -> Relational Operator/2, Add/1, Add1/1, Gain2/1
  Relational Operator/1 -> LiquidIn/1
  Relational Operator1/1 -> LiquidOut/1
  Add/1 -> Add1/2
  Add1/1 -> Relational Operator1/2
  Gain1/1 -> Saturation1/1
  Gain2/1 -> Add/2
  ManualReference/1 -> Gain1/1
  Saturation1/1 -> Relational Operator1/1, Relational Operator/1

== system c00002M_harness/M059/Tank1/Control/ManualControlReference ==
  ManualReference : Inport
  LiquidLevel : Inport  Port=2
  Add : Sum  Inputs=+-
  Add1 : Sum  Inputs=+-
  Gain1 : Gain  Gain=0.95
  Gain2 : Gain  Gain=0.95
  Relational Operator : RelationalOperator  Operator=>  OutDataTypeStr=boolean  RndMeth=Simplest
  Relational Operator1 : RelationalOperator  Operator=<  OutDataTypeStr=boolean  RndMeth=Simplest
  Saturation1 : Saturate  UpperLimit=hmax*0.9  LowerLimit=0
  LiquidIn : Outport
  LiquidOut : Outport  Port=2
  wires:
  LiquidLevel/1 -> Relational Operator/2, Add/1, Add1/1, Gain2/1
  Relational Operator/1 -> LiquidIn/1
  Relational Operator1/1 -> LiquidOut/1
  Add/1 -> Add1/2
  Add1/1 -> Relational Operator1/2
  Gain1/1 -> Saturation1/1
  Gain2/1 -> Add/2
  ManualReference/1 -> Gain1/1
  Saturation1/1 -> Relational Operator1/1, Relational Operator/1

== system c00002M_harness/M059/Tank3/Control/ManualControlReference ==
  ManualReference : Inport
  LiquidLevel : Inport  Port=2
  Add : Sum  Inputs=+-
  Add1 : Sum  Inputs=+-
  Gain1 : Gain  Gain=0.95
  Gain2 : Gain  Gain=0.95
  Relational Operator : RelationalOperator  Operator=>  OutDataTypeStr=boolean  RndMeth=Simplest
  Relational Operator1 : RelationalOperator  Operator=<  OutDataTypeStr=boolean  RndMeth=Simplest
  Saturation1 : Saturate  UpperLimit=hmax*0.9  LowerLimit=0
  LiquidIn : Outport
  LiquidOut : Outport  Port=2
  wires:
  LiquidLevel/1 -> Relational Operator/2, Add/1, Add1/1, Gain2/1
  Relational Operator/1 -> LiquidIn/1
  Relational Operator1/1 -> LiquidOut/1
  Add/1 -> Add1/2
  Add1/1 -> Relational Operator1/2
  Gain1/1 -> Saturation1/1
  Gain2/1 -> Add/2
  ManualReference/1 -> Gain1/1
  Saturation1/1 -> Relational Operator1/1, Relational Operator/1

== system c00002M_harness/M060/Tank1/Control/ManualControlReference ==
  ManualReference : Inport
  LiquidLevel : Inport  Port=2
  Add : Sum  Inputs=+-
  Add1 : Sum  Inputs=+-
  Gain1 : Gain  Gain=0.95
  Gain2 : Gain  Gain=0.95
  Relational Operator : RelationalOperator  Operator=>  OutDataTypeStr=boolean  RndMeth=Simplest
  Relational Operator1 : RelationalOperator  Operator=<  OutDataTypeStr=boolean  RndMeth=Simplest
  Saturation1 : Saturate  UpperLimit=hmax*0.9  LowerLimit=0
  LiquidIn : Outport
  LiquidOut : Outport  Port=2
  wires:
  LiquidLevel/1 -> Relational Operator/2, Add/1, Add1/1, Gain2/1
  Relational Operator/1 -> LiquidIn/1
  Relational Operator1/1 -> LiquidOut/1
  Add/1 -> Add1/2
  Add1/1 -> Relational Operator1/2
  Gain1/1 -> Saturation1/1
  Gain2/1 -> Add/2
  ManualReference/1 -> Gain1/1
  Saturation1/1 -> Relational Operator1/1, Relational Operator/1

== system c00002M_harness/M060/Tank3/Control/ManualControlReference ==
  ManualReference : Inport
  LiquidLevel : Inport  Port=2
  Add : Sum  Inputs=+-
  Add1 : Sum  Inputs=+-
  Gain1 : Gain  Gain=0.95
  Gain2 : Gain  Gain=0.95
  Relational Operator : RelationalOperator  Operator=>  OutDataTypeStr=boolean  RndMeth=Simplest
  Relational Operator1 : RelationalOperator  Operator=<  OutDataTypeStr=boolean  RndMeth=Simplest
  Saturation1 : Saturate  UpperLimit=hmax*0.9  LowerLimit=0
  LiquidIn : Outport
  LiquidOut : Outport  Port=2
  wires:
  LiquidLevel/1 -> Relational Operator/2, Add/1, Add1/1, Gain2/1
  Relational Operator/1 -> LiquidIn/1
  Relational Operator1/1 -> LiquidOut/1
  Add/1 -> Add1/2
  Add1/1 -> Relational Operator1/2
  Gain1/1 -> Saturation1/1
  Gain2/1 -> Add/2
  ManualReference/1 -> Gain1/1
  Saturation1/1 -> Relational Operator1/1, Relational Operator/1

== system c00002M_harness/M061/Tank1/Control/ManualControlReference ==
  ManualReference : Inport
  LiquidLevel : Inport  Port=2
  Add : Sum  Inputs=+-
  Add1 : Sum  Inputs=+-
  Gain1 : Gain  Gain=0.95
  Gain2 : Gain  Gain=0.95
  Relational Operator : RelationalOperator  Operator=>  OutDataTypeStr=boolean  RndMeth=Simplest
  Relational Operator1 : RelationalOperator  Operator=<  OutDataTypeStr=boolean  RndMeth=Simplest
  Saturation1 : Saturate  UpperLimit=hmax*0.9  LowerLimit=0
  LiquidIn : Outport
  LiquidOut : Outport  Port=2
  wires:
  LiquidLevel/1 -> Relational Operator/2, Add/1, Add1/1, Gain2/1
  Relational Operator/1 -> LiquidIn/1
  Relational Operator1/1 -> LiquidOut/1
  Add/1 -> Add1/2
  Add1/1 -> Relational Operator1/2
  Gain1/1 -> Saturation1/1
  Gain2/1 -> Add/2
  ManualReference/1 -> Gain1/1
  Saturation1/1 -> Relational Operator1/1, Relational Operator/1

== system c00002M_harness/M061/Tank3/Control/ManualControlReference ==
  ManualReference : Inport
  LiquidLevel : Inport  Port=2
  Add : Sum  Inputs=+-
  Add1 : Sum  Inputs=+-
  Gain1 : Gain  Gain=0.95
  Gain2 : Gain  Gain=0.95
  Relational Operator : RelationalOperator  Operator=>  OutDataTypeStr=boolean  RndMeth=Simplest
  Relational Operator1 : RelationalOperator  Operator=<  OutDataTypeStr=boolean  RndMeth=Simplest
  Saturation1 : Saturate  UpperLimit=hmax*0.9  LowerLimit=0
  LiquidIn : Outport
  LiquidOut : Outport  Port=2
  wires:
  LiquidLevel/1 -> Relational Operator/2, Add/1, Add1/1, Gain2/1
  Relational Operator/1 -> LiquidIn/1
  Relational Operator1/1 -> LiquidOut/1
  Add/1 -> Add1/2
  Add1/1 -> Relational Operator1/2
  Gain1/1 -> Saturation1/1
  Gain2/1 -> Add/2
  ManualReference/1 -> Gain1/1
  Saturation1/1 -> Relational Operator1/1, Relational Operator/1

== system c00002M_harness/M069/Tank1/Control/ManualControlReference ==
  ManualReference : Inport
  LiquidLevel : Inport  Port=2
  Add : Sum  Inputs=+-
  Add1 : Sum  Inputs=+-
  Gain1 : Gain  Gain=0.95
  Gain2 : Gain  Gain=0.95
  Relational Operator : RelationalOperator  Operator=>  OutDataTypeStr=boolean  RndMeth=Simplest
  Relational Operator1 : RelationalOperator  Operator=<  OutDataTypeStr=boolean  RndMeth=Simplest
  Saturation1 : Saturate  UpperLimit=hmax*0.9  LowerLimit=0
  LiquidIn : Outport
  LiquidOut : Outport  Port=2
  wires:
  LiquidLevel/1 -> Relational Operator/2, Add/1, Add1/1, Gain2/1
  Relational Operator/1 -> LiquidIn/1
  Relational Operator1/1 -> LiquidOut/1
  Add/1 -> Add1/2
  Add1/1 -> Relational Operator1/2
  Gain1/1 -> Saturation1/1
  Gain2/1 -> Add/2
  ManualReference/1 -> Gain1/1
  Saturation1/1 -> Relational Operator1/1, Relational Operator/1

== system c00002M_harness/M069/Tank3/Control/ManualControlReference ==
  ManualReference : Inport
  LiquidLevel : Inport  Port=2
  Add : Sum  Inputs=+-
  Add1 : Sum  Inputs=+-
  Gain1 : Gain  Gain=0.95
  Gain2 : Gain  Gain=0.95
  Relational Operator : RelationalOperator  Operator=>  OutDataTypeStr=boolean  RndMeth=Simplest
  Relational Operator1 : RelationalOperator  Operator=<  OutDataTypeStr=boolean  RndMeth=Simplest
  Saturation1 : Saturate  UpperLimit=hmax*0.9  LowerLimit=0
  LiquidIn : Outport
  LiquidOut : Outport  Port=2
  wires:
  LiquidLevel/1 -> Relational Operator/2, Add/1, Add1/1, Gain2/1
  Relational Operator/1 -> LiquidIn/1
  Relational Operator1/1 -> LiquidOut/1
  Add/1 -> Add1/2
  Add1/1 -> Relational Operator1/2
  Gain1/1 -> Saturation1/1
  Gain2/1 -> Add/2
  ManualReference/1 -> Gain1/1
  Saturation1/1 -> Relational Operator1/1, Relational Operator/1

== system c00002M_harness/M070/Tank1/Control/ManualControlReference ==
  ManualReference : Inport
  LiquidLevel : Inport  Port=2
  Add : Sum  Inputs=+-
  Add1 : Sum  Inputs=+-
  Gain1 : Gain  Gain=0.95
  Gain2 : Gain  Gain=0.95
  Relational Operator : RelationalOperator  Operator=>  OutDataTypeStr=boolean  RndMeth=Simplest
  Relational Operator1 : RelationalOperator  Operator=<  OutDataTypeStr=boolean  RndMeth=Simplest
  Saturation1 : Saturate  UpperLimit=hmax*0.9  LowerLimit=0
  LiquidIn : Outport
  LiquidOut : Outport  Port=2
  wires:
  LiquidLevel/1 -> Relational Operator/2, Add/1, Add1/1, Gain2/1
  Relational Operator/1 -> LiquidIn/1
  Relational Operator1/1 -> LiquidOut/1
  Add/1 -> Add1/2
  Add1/1 -> Relational Operator1/2
  Gain1/1 -> Saturation1/1
  Gain2/1 -> Add/2
  ManualReference/1 -> Gain1/1
  Saturation1/1 -> Relational Operator1/1, Relational Operator/1

== system c00002M_harness/M070/Tank3/Control/ManualControlReference ==
  ManualReference : Inport
  LiquidLevel : Inport  Port=2
  Add : Sum  Inputs=+-
  Add1 : Sum  Inputs=+-
  Gain1 : Gain  Gain=0.95
  Gain2 : Gain  Gain=0.95
  Relational Operator : RelationalOperator  Operator=>  OutDataTypeStr=boolean  RndMeth=Simplest
  Relational Operator1 : RelationalOperator  Operator=<  OutDataTypeStr=boolean  RndMeth=Simplest
  Saturation1 : Saturate  UpperLimit=hmax*0.9  LowerLimit=0
  LiquidIn : Outport
  LiquidOut : Outport  Port=2
  wires:
  LiquidLevel/1 -> Relational Operator/2, Add/1, Add1/1, Gain2/1
  Relational Operator/1 -> LiquidIn/1
  Relational Operator1/1 -> LiquidOut/1
  Add/1 -> Add1/2
  Add1/1 -> Relational Operator1/2
  Gain1/1 -> Saturation1/1
  Gain2/1 -> Add/2
  ManualReference/1 -> Gain1/1
  Saturation1/1 -> Relational Operator1/1, Relational Operator/1

== system c00002M_harness/M071/Tank1/Control/ManualControlReference ==
  ManualReference : Inport
  LiquidLevel : Inport  Port=2
  Add : Sum  Inputs=+-
  Add1 : Sum  Inputs=+-
  Gain1 : Gain  Gain=0.95
  Gain2 : Gain  Gain=0.95
  Relational Operator : RelationalOperator  Operator=>  OutDataTypeStr=boolean  RndMeth=Simplest
  Relational Operator1 : RelationalOperator  Operator=<  OutDataTypeStr=boolean  RndMeth=Simplest
  Saturation1 : Saturate  UpperLimit=hmax*0.9  LowerLimit=0
  LiquidIn : Outport
  LiquidOut : Outport  Port=2
  wires:
  LiquidLevel/1 -> Relational Operator/2, Add/1, Add1/1, Gain2/1
  Relational Operator/1 -> LiquidIn/1
  Relational Operator1/1 -> LiquidOut/1
  Add/1 -> Add1/2
  Add1/1 -> Relational Operator1/2
  Gain1/1 -> Saturation1/1
  Gain2/1 -> Add/2
  ManualReference/1 -> Gain1/1
  Saturation1/1 -> Relational Operator1/1, Relational Operator/1

== system c00002M_harness/M071/Tank3/Control/ManualControlReference ==
  ManualReference : Inport
  LiquidLevel : Inport  Port=2
  Add : Sum  Inputs=+-
  Add1 : Sum  Inputs=+-
  Gain1 : Gain  Gain=0.95
  Gain2 : Gain  Gain=0.95
  Relational Operator : RelationalOperator  Operator=>  OutDataTypeStr=boolean  RndMeth=Simplest
  Relational Operator1 : RelationalOperator  Operator=<  OutDataTypeStr=boolean  RndMeth=Simplest
  Saturation1 : Saturate  UpperLimit=hmax*0.9  LowerLimit=0
  LiquidIn : Outport
  LiquidOut : Outport  Port=2
  wires:
  LiquidLevel/1 -> Relational Operator/2, Add/1, Add1/1, Gain2/1
  Relational Operator/1 -> LiquidIn/1
  Relational Operator1/1 -> LiquidOut/1
  Add/1 -> Add1/2
  Add1/1 -> Relational Operator1/2
  Gain1/1 -> Saturation1/1
  Gain2/1 -> Add/2
  ManualReference/1 -> Gain1/1
  Saturation1/1 -> Relational Operator1/1, Relational Operator/1

== system c00002M_harness/M072/Tank1/Control/ManualControlReference ==
  ManualReference : Inport
  LiquidLevel : Inport  Port=2
  Add : Sum  Inputs=+-
  Add1 : Sum  Inputs=+-
  Gain1 : Gain  Gain=0.95
  Gain2 : Gain  Gain=0.95
  Relational Operator : RelationalOperator  Operator=>  OutDataTypeStr=boolean  RndMeth=Simplest
  Relational Operator1 : RelationalOperator  Operator=<  OutDataTypeStr=boolean  RndMeth=Simplest
  Saturation1 : Saturate  UpperLimit=hmax*0.9  LowerLimit=0
  LiquidIn : Outport
  LiquidOut : Outport  Port=2
  wires:
  LiquidLevel/1 -> Relational Operator/2, Add/1, Add1/1, Gain2/1
  Relational Operator/1 -> LiquidIn/1
  Relational Operator1/1 -> LiquidOut/1
  Add/1 -> Add1/2
  Add1/1 -> Relational Operator1/2
  Gain1/1 -> Saturation1/1
  Gain2/1 -> Add/2
  ManualReference/1 -> Gain1/1
  Saturation1/1 -> Relational Operator1/1, Relational Operator/1

== system c00002M_harness/M072/Tank3/Control/ManualControlReference ==
  ManualReference : Inport
  LiquidLevel : Inport  Port=2
  Add : Sum  Inputs=+-
  Add1 : Sum  Inputs=+-
  Gain1 : Gain  Gain=0.95
  Gain2 : Gain  Gain=0.95
  Relational Operator : RelationalOperator  Operator=>  OutDataTypeStr=boolean  RndMeth=Simplest
  Relational Operator1 : RelationalOperator  Operator=<  OutDataTypeStr=boolean  RndMeth=Simplest
  Saturation1 : Saturate  UpperLimit=hmax*0.9  LowerLimit=0
  LiquidIn : Outport
  LiquidOut : Outport  Port=2
  wires:
  LiquidLevel/1 -> Relational Operator/2, Add/1, Add1/1, Gain2/1
  Relational Operator/1 -> LiquidIn/1
  Relational Operator1/1 -> LiquidOut/1
  Add/1 -> Add1/2
  Add1/1 -> Relational Operator1/2
  Gain1/1 -> Saturation1/1
  Gain2/1 -> Add/2
  ManualReference/1 -> Gain1/1
  Saturation1/1 -> Relational Operator1/1, Relational Operator/1

== system c00002M_harness/M073/Tank1/Control/ManualControlReference ==
  ManualReference : Inport
  LiquidLevel : Inport  Port=2
  Add : Sum  Inputs=+-
  Add1 : Sum  Inputs=+-
  Gain1 : Gain  Gain=0.95
  Gain2 : Gain  Gain=0.95
  Relational Operator : RelationalOperator  Operator=>  OutDataTypeStr=boolean  RndMeth=Simplest
  Relational Operator1 : RelationalOperator  Operator=<  OutDataTypeStr=boolean  RndMeth=Simplest
  Saturation1 : Saturate  UpperLimit=hmax*0.9  LowerLimit=0
  LiquidIn : Outport
  LiquidOut : Outport  Port=2
  wires:
  LiquidLevel/1 -> Relational Operator/2, Add/1, Add1/1, Gain2/1
  Relational Operator/1 -> LiquidIn/1
  Relational Operator1/1 -> LiquidOut/1
  Add/1 -> Add1/2
  Add1/1 -> Relational Operator1/2
  Gain1/1 -> Saturation1/1
  Gain2/1 -> Add/2
  ManualReference/1 -> Gain1/1
  Saturation1/1 -> Relational Operator1/1, Relational Operator/1

== system c00002M_harness/M073/Tank3/Control/ManualControlReference ==
  ManualReference : Inport
  LiquidLevel : Inport  Port=2
  Add : Sum  Inputs=+-
  Add1 : Sum  Inputs=+-
  Gain1 : Gain  Gain=0.95
  Gain2 : Gain  Gain=0.95
  Relational Operator : RelationalOperator  Operator=>  OutDataTypeStr=boolean  RndMeth=Simplest
  Relational Operator1 : RelationalOperator  Operator=<  OutDataTypeStr=boolean  RndMeth=Simplest
  Saturation1 : Saturate  UpperLimit=hmax*0.9  LowerLimit=0
  LiquidIn : Outport
  LiquidOut : Outport  Port=2
  wires:
  LiquidLevel/1 -> Relational Operator/2, Add/1, Add1/1, Gain2/1
  Relational Operator/1 -> LiquidIn/1
  Relational Operator1/1 -> LiquidOut/1
  Add/1 -> Add1/2
  Add1/1 -> Relational Operator1/2
  Gain1/1 -> Saturation1/1
  Gain2/1 -> Add/2
  ManualReference/1 -> Gain1/1
  Saturation1/1 -> Relational Operator1/1, Relational Operator/1

== system c00002M_harness/M074/Tank1/Control/ManualControlReference ==
  ManualReference : Inport
  LiquidLevel : Inport  Port=2
  Add : Sum  Inputs=+-
  Add1 : Sum  Inputs=+-
  Gain1 : Gain  Gain=0.95
  Gain2 : Gain  Gain=0.95
  Relational Operator : RelationalOperator  Operator=>  OutDataTypeStr=boolean  RndMeth=Simplest
  Relational Operator1 : RelationalOperator  Operator=<  OutDataTypeStr=boolean  RndMeth=Simplest
  Saturation1 : Saturate  UpperLimit=hmax*0.9  LowerLimit=0
  LiquidIn : Outport
  LiquidOut : Outport  Port=2
  wires:
  LiquidLevel/1 -> Relational Operator/2, Add/1, Add1/1, Gain2/1
  Relational Operator/1 -> LiquidIn/1
  Relational Operator1/1 -> LiquidOut/1
  Add/1 -> Add1/2
  Add1/1 -> Relational Operator1/2
  Gain1/1 -> Saturation1/1
  Gain2/1 -> Add/2
  ManualReference/1 -> Gain1/1
  Saturation1/1 -> Relational Operator1/1, Relational Operator/1
